simulink model "ExtIOTop"  (R2015a)
settings: Solver=FixedStepDiscrete  StartTime=0.0  StopTime=10.0  FixedStep=0.01  RelTol=1e-3
settings Model: Creator=mbd_user  LastModifiedBy=mbd_user

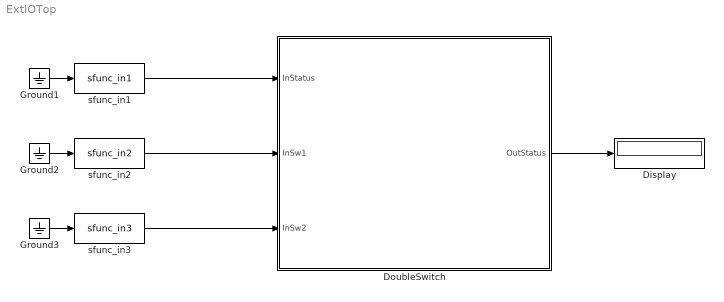
== system ExtIOTop ==
  Display : Display
  DoubleSwitch : Subsystem  TreatAsAtomicUnit=on
  Ground1 : Ground
  Ground2 : Ground
  Ground3 : Ground
  sfunc_in1 : MATLABFcn  MATLABFcn=sfunc_in1
  sfunc_in2 : MATLABFcn  MATLABFcn=sfunc_in2
  sfunc_in3 : MATLABFcn  MATLABFcn=sfunc_in3
  wires:
  Ground1/1 -> sfunc_in1/1
  Ground2/1 -> sfunc_in2/1
  Ground3/1 -> sfunc_in3/1
  DoubleSwitch/1(OutStatus) -> Display/1
  sfunc_in2/1 -> DoubleSwitch/2(InSw1)
  sfunc_in3/1 -> DoubleSwitch/3(InSw2)
  sfunc_in1/1 -> DoubleSwitch/1(InStatus)

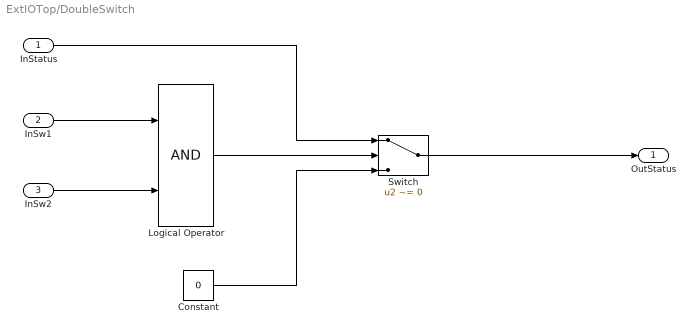
== system ExtIOTop/DoubleSwitch ==
  InStatus : Inport
  InSw1 : Inport  Port=2
  InSw2 : Inport  Port=3
  Constant : Constant  Value=0
  Logical Operator : Logic  AllPortsSameDT=off  OutDataTypeStr=boolean
  Switch : Switch  Criteria=u2 ~= 0
  OutStatus : Outport
  wires:
  InSw1/1 -> Logical Operator/1
  InSw2/1 -> Logical Operator/2
  Logical Operator/1 -> Switch/2
  InStatus/1 -> Switch/1
  Switch/1 -> OutStatus/1
  Constant/1 -> Switch/3
